simulink model "Aufgabe10_Teilsysteme"  (R2022a)
settings: Solver=ode3  StartTime=0.0  StopTime=80  FixedStep=0.01  RelTol=1e-3
undefined symbols (not defined in the file): A, I, igetr, K, MRK, PHI, Ra, sigbuilder_block, U
libraries: simulink x25
settings Model: Creator=60251  LastModifiedBy=60251

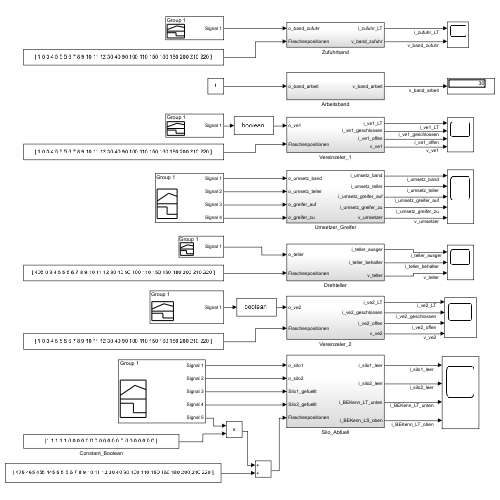
[thumbnail: Simulink's stored preview of the top-level diagram]
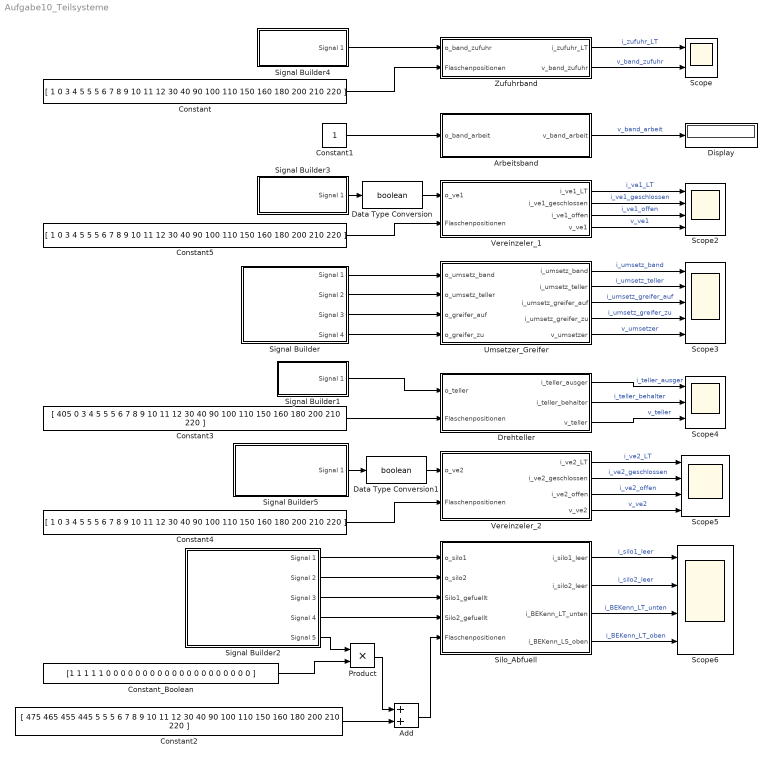
== system Aufgabe10_Teilsysteme ==
  Add : Sum
  Arbeitsband : Subsystem
  Constant : Constant  Value=[ 1 0 3 4 5 5 5 6 7 8 9 10 11 12 30 40 90 100 110 150 160 180 200 210 220 ]
  Constant1 : Constant
  Constant2 : Constant  Value=[ 475 465 455 445 5 5 5 6 7 8 9 10 11 12 30 40 90 100 110 150 160 180 200 210 220 ]
  Constant3 : Constant  Value=[ 405 0 3 4 5 5 5 6 7 8 9 10 11 12 30 40 90 100 110 150 160 180 200 210 220 ]
  Constant4 : Constant  Value=[ 1 0 3 4 5 5 5 6 7 8 9 10 11 12 30 40 90 100 110 150 160 180 200 210 220 ]
  Constant5 : Constant  Value=[ 1 0 3 4 5 5 5 6 7 8 9 10 11 12 30 40 90 100 110 150 160 180 200 210 220 ]
  Constant_Boolean : Constant  Value=[1 1 1 1 1 0 0 0 0 0 0 0 0 0 0 0 0 0 0 0 0 0 0 0 0 ]
  Data Type Conversion : DataTypeConversion  OutDataTypeStr=boolean  SaturateOnIntegerOverflow=off  RndMeth=Floor
  Data Type Conversion1 : DataTypeConversion  OutDataTypeStr=boolean  SaturateOnIntegerOverflow=off  RndMeth=Floor
  Display : Display
  Drehteller : Subsystem
  Product : Product
  Scope : Scope  NumInputPorts=2
  Scope2 : Scope  NumInputPorts=4
  Scope3 : Scope  NumInputPorts=5
  Scope4 : Scope  NumInputPorts=3
  Scope5 : Scope  NumInputPorts=4
  Scope6 : Scope  NumInputPorts=4
  Signal Builder : Subsystem  Tag=STV Subsys  LoadFcn=sigbuilder_block('load');  StartFcn=sigbuilder_block('start');  StopFcn=sigbuilder_block('stop');  ClipboardFcn=sigbuilder_block('clipboard');  mask(Sigbuilder block){tuvar=[0:10]}
      mask help: Simulink:masks:SigbuilderBlock_MD
      mask init:
      | if ~strcmp(get_param(bdroot(gcbh),'SimulationStatus'),'stopped') tuvar = sigbuilder_block('maskInit'); end
      settings: CopyFcn=sigbuilder_block('copy');  DeleteFcn=sigbuilder_block('delete');  ModelCloseFcn=sigbuilder_block('modelClose');  PreSaveFcn=sigbuilder_block('preSave');  PauseFcn=sigbuilder_block('pause');  ContinueFcn=sigbuilder_block('continue');  NameChangeFcn=sigbuilder_block('namechange');  OpenFcn=sigbuilder_block('open',[217.2 175.2 488.4 312 ]);  CloseFcn=sigbuilder_block('close');
      mask Display: plot(0, 0, 100, 100,[2, 2, 32, 32, 2], [68, 8, 8, 68, 68],[32, 2], [38, 38], [32, 19, 2],[53, 60, 44], [32, 17, 17, 2],[16, 16, 31, 31]);txt = getActiveGroup(gcbh);text(2, 100, txt,'verticalAlignment', 'top');
  Signal Builder1 : Subsystem  Tag=STV Subsys  LoadFcn=sigbuilder_block('load');  StartFcn=sigbuilder_block('start');  StopFcn=sigbuilder_block('stop');  ClipboardFcn=sigbuilder_block('clipboard');  mask(Sigbuilder block){tuvar=[0:10]}
      mask help: Simulink:masks:SigbuilderBlock_MD
      mask init:
      | if ~strcmp(get_param(bdroot(gcbh),'SimulationStatus'),'stopped') tuvar = sigbuilder_block('maskInit'); end
      settings: CopyFcn=sigbuilder_block('copy');  DeleteFcn=sigbuilder_block('delete');  ModelCloseFcn=sigbuilder_block('modelClose');  PreSaveFcn=sigbuilder_block('preSave');  PauseFcn=sigbuilder_block('pause');  ContinueFcn=sigbuilder_block('continue');  NameChangeFcn=sigbuilder_block('namechange');  OpenFcn=sigbuilder_block('open',[279 117 550.8 361.8 ]);  CloseFcn=sigbuilder_block('close');
      mask Display: plot(0, 0, 100, 100,[2, 2, 32, 32, 2], [68, 8, 8, 68, 68],[32, 2], [38, 38], [32, 19, 2],[53, 60, 44], [32, 17, 17, 2],[16, 16, 31, 31]);txt = getActiveGroup(gcbh);text(2, 100, txt,'verticalAlignment', 'top');
  Signal Builder2 : Subsystem  Tag=STV Subsys  LoadFcn=sigbuilder_block('load');  StartFcn=sigbuilder_block('start');  StopFcn=sigbuilder_block('stop');  ClipboardFcn=sigbuilder_block('clipboard');  mask(Sigbuilder block){tuvar=[0:10]}
      mask help: Simulink:masks:SigbuilderBlock_MD
      mask init:
      | if ~strcmp(get_param(bdroot(gcbh),'SimulationStatus'),'stopped') tuvar = sigbuilder_block('maskInit'); end
      settings: CopyFcn=sigbuilder_block('copy');  DeleteFcn=sigbuilder_block('delete');  ModelCloseFcn=sigbuilder_block('modelClose');  PreSaveFcn=sigbuilder_block('preSave');  PauseFcn=sigbuilder_block('pause');  ContinueFcn=sigbuilder_block('continue');  NameChangeFcn=sigbuilder_block('namechange');  OpenFcn=sigbuilder_block('open',[61.5 156.75 659.25 447 ]);  CloseFcn=sigbuilder_block('close');
      mask Display: plot(0, 0, 100, 100,[2, 2, 32, 32, 2], [68, 8, 8, 68, 68],[32, 2], [38, 38], [32, 19, 2],[53, 60, 44], [32, 17, 17, 2],[16, 16, 31, 31]);txt = getActiveGroup(gcbh);text(2, 100, txt,'verticalAlignment', 'top');
  Signal Builder3 : Subsystem  Tag=STV Subsys  LoadFcn=sigbuilder_block('load');  StartFcn=sigbuilder_block('start');  StopFcn=sigbuilder_block('stop');  ClipboardFcn=sigbuilder_block('clipboard');  mask(Sigbuilder block){tuvar=[0:10]}
      mask help: Simulink:masks:SigbuilderBlock_MD
      mask init:
      | if ~strcmp(get_param(bdroot(gcbh),'SimulationStatus'),'stopped') tuvar = sigbuilder_block('maskInit'); end
      settings: CopyFcn=sigbuilder_block('copy');  DeleteFcn=sigbuilder_block('delete');  ModelCloseFcn=sigbuilder_block('modelClose');  PreSaveFcn=sigbuilder_block('preSave');  PauseFcn=sigbuilder_block('pause');  ContinueFcn=sigbuilder_block('continue');  NameChangeFcn=sigbuilder_block('namechange');  OpenFcn=sigbuilder_block('open',[30.75 168 550.5 396 ]);  CloseFcn=sigbuilder_block('close');
      mask Display: plot(0, 0, 100, 100,[2, 2, 32, 32, 2], [68, 8, 8, 68, 68],[32, 2], [38, 38], [32, 19, 2],[53, 60, 44], [32, 17, 17, 2],[16, 16, 31, 31]);txt = getActiveGroup(gcbh);text(2, 100, txt,'verticalAlignment', 'top');
  Signal Builder4 : Subsystem  Tag=STV Subsys  LoadFcn=sigbuilder_block('load');  StartFcn=sigbuilder_block('start');  StopFcn=sigbuilder_block('stop');  ClipboardFcn=sigbuilder_block('clipboard');  mask(Sigbuilder block){tuvar=[0:10]}
      mask help: Simulink:masks:SigbuilderBlock_MD
      mask init:
      | if ~strcmp(get_param(bdroot(gcbh),'SimulationStatus'),'stopped') tuvar = sigbuilder_block('maskInit'); end
      settings: CopyFcn=sigbuilder_block('copy');  DeleteFcn=sigbuilder_block('delete');  ModelCloseFcn=sigbuilder_block('modelClose');  PreSaveFcn=sigbuilder_block('preSave');  PauseFcn=sigbuilder_block('pause');  ContinueFcn=sigbuilder_block('continue');  NameChangeFcn=sigbuilder_block('namechange');  OpenFcn=sigbuilder_block('open',[225.6 94.2 550.8 321 ]);  CloseFcn=sigbuilder_block('close');
      mask Display: plot(0, 0, 100, 100,[2, 2, 32, 32, 2], [68, 8, 8, 68, 68],[32, 2], [38, 38], [32, 19, 2],[53, 60, 44], [32, 17, 17, 2],[16, 16, 31, 31]);txt = getActiveGroup(gcbh);text(2, 100, txt,'verticalAlignment', 'top');
  Signal Builder5 : Subsystem  Tag=STV Subsys  LoadFcn=sigbuilder_block('load');  StartFcn=sigbuilder_block('start');  StopFcn=sigbuilder_block('stop');  ClipboardFcn=sigbuilder_block('clipboard');  mask(Sigbuilder block){tuvar=[0:10]}
      mask help: Simulink:masks:SigbuilderBlock_MD
      mask init:
      | if ~strcmp(get_param(bdroot(gcbh),'SimulationStatus'),'stopped') tuvar = sigbuilder_block('maskInit'); end
      settings: CopyFcn=sigbuilder_block('copy');  DeleteFcn=sigbuilder_block('delete');  ModelCloseFcn=sigbuilder_block('modelClose');  PreSaveFcn=sigbuilder_block('preSave');  PauseFcn=sigbuilder_block('pause');  ContinueFcn=sigbuilder_block('continue');  NameChangeFcn=sigbuilder_block('namechange');  OpenFcn=sigbuilder_block('open',[46.5 97.5 550.5 399.75 ]);  CloseFcn=sigbuilder_block('close');
      mask Display: plot(0, 0, 100, 100,[2, 2, 32, 32, 2], [68, 8, 8, 68, 68],[32, 2], [38, 38], [32, 19, 2],[53, 60, 44], [32, 17, 17, 2],[16, 16, 31, 31]);txt = getActiveGroup(gcbh);text(2, 100, txt,'verticalAlignment', 'top');
  Silo_Abfuell : Subsystem
  Umsetzer_Greifer : Subsystem
  Vereinzeler_1 : Subsystem
  Vereinzeler_2 : Subsystem
  Zufuhrband : Subsystem
  wires:
  Signal Builder4/1(Signal 1) -> Zufuhrband/1(o_band_zufuhr)
  Constant/1 -> Zufuhrband/2(Flaschenpositionen)
  Zufuhrband/1(i_zufuhr_LT) -> Scope/1  "i_zufuhr_LT"
  Zufuhrband/2(v_band_zufuhr) -> Scope/2  "v_band_zufuhr"
  Constant1/1 -> Arbeitsband/1(o_band_arbeit)
  Arbeitsband/1(v_band_arbeit) -> Display/1  "v_band_arbeit"
  Signal Builder3/1(Signal 1) -> Data Type Conversion/1
  Data Type Conversion/1 -> Vereinzeler_1/1(o_ve1)
  Constant5/1 -> Vereinzeler_1/2(Flaschenpositionen)
  Vereinzeler_1/1(i_ve1_LT) -> Scope2/1  "i_ve1_LT"
  Vereinzeler_1/2(i_ve1_geschlossen) -> Scope2/2  "i_ve1_geschlossen"
  Vereinzeler_1/3(i_ve1_offen) -> Scope2/3  "i_ve1_offen"
  Vereinzeler_1/4(v_ve1) -> Scope2/4  "v_ve1"
  Signal Builder/1(Signal 1) -> Umsetzer_Greifer/1(o_umsetz_band)
  Signal Builder/2(Signal 2) -> Umsetzer_Greifer/2(o_umsetz_teller)
  Signal Builder/3(Signal 3) -> Umsetzer_Greifer/3(o_greifer_auf)
  Signal Builder/4(Signal 4) -> Umsetzer_Greifer/4(o_greifer_zu)
  Umsetzer_Greifer/3(i_umsetz_greifer_auf) -> Scope3/3  "i_umsetz_greifer_auf"
  Umsetzer_Greifer/2(i_umsetz_teller) -> Scope3/2  "i_umsetz_teller"
  Umsetzer_Greifer/4(i_umsetz_greifer_zu) -> Scope3/4  "i_umsetz_greifer_zu"
  Umsetzer_Greifer/1(i_umsetz_band) -> Scope3/1  "i_umsetz_band"
  Umsetzer_Greifer/5(v_umsetzer) -> Scope3/5  "v_umsetzer"
  Drehteller/2(i_teller_behalter) -> Scope4/2  "i_teller_behalter"
  Drehteller/1(i_teller_ausger) -> Scope4/1  "i_teller_ausger"
  Drehteller/3(v_teller) -> Scope4/3  "v_teller"
  Constant3/1 -> Drehteller/2(Flaschenpositionen)
  Signal Builder1/1(Signal 1) -> Drehteller/1(o_teller)
  Vereinzeler_2/2(i_ve2_geschlossen) -> Scope5/2  "i_ve2_geschlossen"
  Vereinzeler_2/1(i_ve2_LT) -> Scope5/1  "i_ve2_LT"
  Vereinzeler_2/3(i_ve2_offen) -> Scope5/3  "i_ve2_offen"
  Vereinzeler_2/4(v_ve2) -> Scope5/4  "v_ve2"
  Signal Builder5/1(Signal 1) -> Data Type Conversion1/1
  Constant4/1 -> Vereinzeler_2/2(Flaschenpositionen)
  Data Type Conversion1/1 -> Vereinzeler_2/1(o_ve2)
  Silo_Abfuell/1(i_silo1_leer) -> Scope6/1  "i_silo1_leer"
  Silo_Abfuell/2(i_silo2_leer) -> Scope6/2  "i_silo2_leer"
  Silo_Abfuell/3(i_BEKenn_LT_unten) -> Scope6/3  "i_BEKenn_LT_unten"
  Silo_Abfuell/4(i_BEKenn_LS_oben) -> Scope6/4  "i_BEKenn_LT_oben"
  Signal Builder2/5(Signal 5) -> Product/1
  Constant_Boolean/1 -> Product/2
  Product/1 -> Add/1
  Constant2/1 -> Add/2
  Add/1 -> Silo_Abfuell/5(Flaschenpositionen)
  Signal Builder2/1(Signal 1) -> Silo_Abfuell/1(o_silo1)
  Signal Builder2/2(Signal 2) -> Silo_Abfuell/2(o_silo2)
  Signal Builder2/3(Signal 3) -> Silo_Abfuell/3(Silo1_gefuellt)
  Signal Builder2/4(Signal 4) -> Silo_Abfuell/4(Silo2_gefuellt)

== system Aufgabe10_Teilsysteme/Arbeitsband ==
  o_band_arbeit : Inport
  Gain : Gain  Gain=30
  v_band_arbeit : Outport
  wires:
  o_band_arbeit/1 -> Gain/1
  Gain/1 -> v_band_arbeit/1

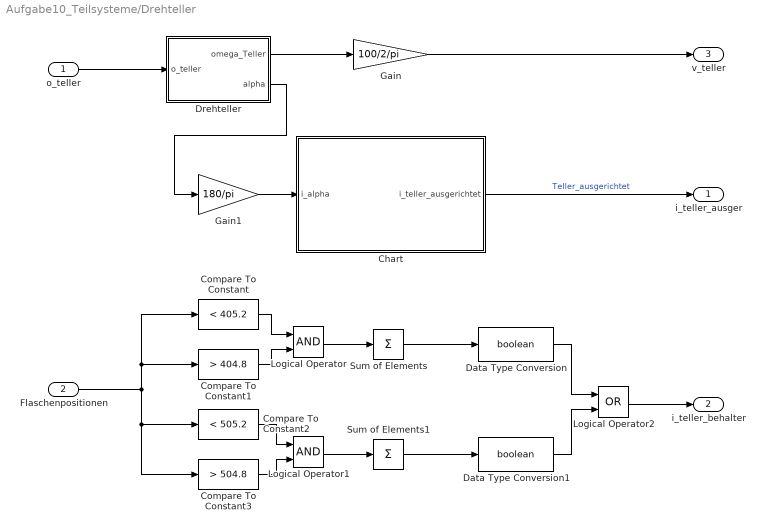
== system Aufgabe10_Teilsysteme/Drehteller ==
  o_teller : Inport
  Flaschenpositionen : Inport  Port=2
  Chart : Stateflow chart  TreatAsAtomicUnit=on
  Compare To Constant : simulink/Logic and Bit Operations/Compare To Constant  relop=<  const=405.2  OutDataTypeStr=boolean
  Compare To Constant1 : simulink/Logic and Bit Operations/Compare To Constant  relop=>  const=404.8  OutDataTypeStr=boolean
  Compare To Constant2 : simulink/Logic and Bit Operations/Compare To Constant  relop=<  const=505.2  OutDataTypeStr=boolean
  Compare To Constant3 : simulink/Logic and Bit Operations/Compare To Constant  relop=>  const=504.8  OutDataTypeStr=boolean
  Data Type Conversion : DataTypeConversion  OutDataTypeStr=boolean  SaturateOnIntegerOverflow=off  RndMeth=Floor
  Data Type Conversion1 : DataTypeConversion  OutDataTypeStr=boolean  SaturateOnIntegerOverflow=off  RndMeth=Floor
  Drehteller : Subsystem
  Gain : Gain  Gain=100/2/pi
  Gain1 : Gain  Gain=180/pi
  Logical Operator : Logic  AllPortsSameDT=off  OutDataTypeStr=boolean
  Logical Operator1 : Logic  AllPortsSameDT=off  OutDataTypeStr=boolean
  Logical Operator2 : Logic  Operator=OR  AllPortsSameDT=off  OutDataTypeStr=boolean
  Sum of Elements : Sum  Inputs=+
  Sum of Elements1 : Sum  Inputs=+
  i_teller_ausger : Outport
  i_teller_behalter : Outport  Port=2
  v_teller : Outport  Port=3
  wires:
  Compare To Constant/1 -> Logical Operator/1
  Compare To Constant1/1 -> Logical Operator/2
  Compare To Constant2/1 -> Logical Operator1/1
  Compare To Constant3/1 -> Logical Operator1/2
  Logical Operator/1 -> Sum of Elements/1
  Logical Operator1/1 -> Sum of Elements1/1
  Sum of Elements1/1 -> Data Type Conversion1/1
  Sum of Elements/1 -> Data Type Conversion/1
  Flaschenpositionen/1 -> Compare To Constant3/1, Compare To Constant2/1, Compare To Constant/1, Compare To Constant1/1
  Data Type Conversion/1 -> Logical Operator2/1
  Data Type Conversion1/1 -> Logical Operator2/2
  Logical Operator2/1 -> i_teller_behalter/1
  o_teller/1 -> Drehteller/1(o_teller)
  Drehteller/1(omega_Teller) -> Gain/1
  Gain/1 -> v_teller/1
  Chart/1(i_teller_ausgerichtet) -> i_teller_ausger/1  "Teller_ausgerichtet"
  Gain1/1 -> Chart/1(i_alpha)
  Drehteller/2(alpha) -> Gain1/1

== system Aufgabe10_Teilsysteme/Signal Builder ==
  Demux : Demux  Tag=STV Demux
      settings: DisplayOption=none
  FromWs : FromWorkspace  Tag=STV FromWs  VariableName=tuvar
      SigBuilderData=|
      | common.afterFinalStr = 'Extrapolate'
      | common.sampleTime = 0
      | dataSet.timeRange = [0 50]
      | dataSet.name = 'Group 1'
      | sbobj.Groups.Name = 'Group 1'
      | sbobj.Groups.Signals(1).Name = 'Signal 1'
      | sbobj.Groups.Signals(1).XData = [0 2 2 8 8 20.1 25 50]
      | sbobj.Groups.Signals(1).YData = [0 0 1 1 0 0 0 0]
      | sbobj.Groups.Signals(2).Name = 'Signal 2'
      | sbobj.Groups.Signals(2).XData = [0 4 5.7 5.7 7.2 7.2 20.1 20.1 25 25 50]
      | sbobj.Groups.Signals(2).YData = [0 0 0 1 1 0 0 1 1 0 0]
      | sbobj.Groups.Signals(3).Name = 'Signal 3'
      | sbobj.Groups.Signals(3).XData = [0 3 3 3.2 3.2 6 10 10 10.8 10.8 30 30 31.5 31.5 50]
      | sbobj.Groups.Signals(3).YData = [0 0 1 1 0 0 0 1 1 0 0 1 1 0 0]
      | sbobj.Groups.Signals(4).Name = 'Signal 4'
      | sbobj.Groups.Signals(4).XData = [0 4 4 5 5 6 13.7 13.7 15 15 30 30 31.5 31.5 50]
      | sbobj.Groups.Signals(4).YData = [0 0 1 1 0 0 0 1 1 0 0 1 1 0 0]
      | sbobj.Groups.TimeRange = [0 50]
  Signal 1 : Outport  Tag=STV Outport  VectorParamsAs1DForOutWhenUnconnected=off
  Signal 2 : Outport  Tag=STV Outport  Port=2  VectorParamsAs1DForOutWhenUnconnected=off
  Signal 3 : Outport  Tag=STV Outport  Port=3  VectorParamsAs1DForOutWhenUnconnected=off
  Signal 4 : Outport  Tag=STV Outport  Port=4  VectorParamsAs1DForOutWhenUnconnected=off
  wires:
  Demux/1 -> Signal 1/1
  FromWs/1 -> Demux/1
  Demux/2 -> Signal 2/1
  Demux/3 -> Signal 3/1
  Demux/4 -> Signal 4/1

== system Aufgabe10_Teilsysteme/Signal Builder1 ==
  Demux : Demux  Tag=STV Demux  Outputs=1
      settings: DisplayOption=none
  FromWs : FromWorkspace  Tag=STV FromWs  VariableName=tuvar
      SigBuilderData=|
      | common.afterFinalStr = 'Extrapolate'
      | common.sampleTime = 0
      | dataSet.timeRange = [0 50]
      | dataSet.name = 'Group 1'
      | sbobj.Groups.Name = 'Group 1'
      | sbobj.Groups.Signals.Name = 'Signal 1'
      | sbobj.Groups.Signals.XData = [0 1 1 4 6 30 30 40 40 50]
      | sbobj.Groups.Signals.YData = [0 0 1 1 1 1 0 0 1 1]
      | sbobj.Groups.TimeRange = [0 50]
  Signal 1 : Outport  Tag=STV Outport  VectorParamsAs1DForOutWhenUnconnected=off
  wires:
  Demux/1 -> Signal 1/1
  FromWs/1 -> Demux/1

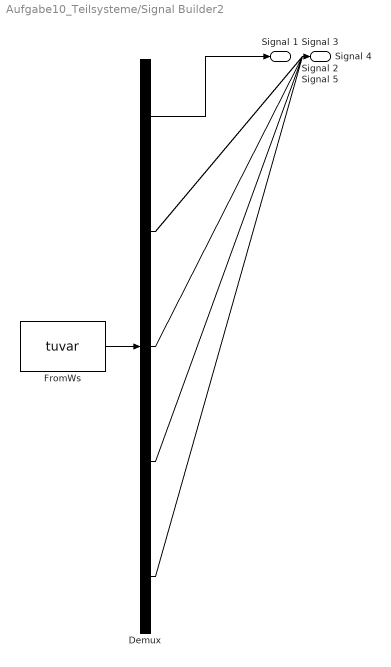
== system Aufgabe10_Teilsysteme/Signal Builder2 ==
  Demux : Demux  Tag=STV Demux  Outputs=5
      settings: DisplayOption=none
  FromWs : FromWorkspace  Tag=STV FromWs  VariableName=tuvar
      SigBuilderData=|
      | common.afterFinalStr = 'Extrapolate'
      | common.sampleTime = 0
      | dataSet.timeRange = [0 80]
      | dataSet.name = 'Group 1'
      | sbobj.Groups.Name = 'Group 1'
      | sbobj.Groups.Signals(1).Name = 'Signal 1'
      | sbobj.Groups.Signals(1).XData = [0 1 1 4 6 6 21.5 21.5 31 31 40 40 60 60 80]
      | sbobj.Groups.Signals(1).YData = [0 0 1 1 1 0 0 1 1 0 0 1 1 0 0]
      | sbobj.Groups.Signals(2).Name = 'Signal 2'
      | sbobj.Groups.Signals(2).XData = [0 1 1 6 6 40 80]
      | sbobj.Groups.Signals(2).YData = [0 0 1 1 0 0 0]
      | sbobj.Groups.Signals(3).Name = 'Signal 3'
      | sbobj.Groups.Signals(3).XData = [0 35 35 40.5 40.5 50 59.5 80]
      | sbobj.Groups.Signals(3).YData = [0 0 1 1 0 0 0 0]
      | sbobj.Groups.Signals(4).Name = 'Signal 4'
      | sbobj.Groups.Signals(4).XData = [0 50 60 80]
      | sbobj.Groups.Signals(4).YData = [0 0 0 0]
      | sbobj.Groups.Signals(5).Name = 'Signal 5'
      | sbobj.Groups.Signals(5).XData = [0 1 1 14.8 14.8 20 20 35 35 40 40 80]
      | sbobj.Groups.Signals(5).YData = [0 0 5 5 10 10 15 15 20 20 25 25]
      | sbobj.Groups.TimeRange = [0 80]
  Signal 1 : Outport  Tag=STV Outport  VectorParamsAs1DForOutWhenUnconnected=off
  Signal 2 : Outport  Tag=STV Outport  Port=2  VectorParamsAs1DForOutWhenUnconnected=off
  Signal 3 : Outport  Tag=STV Outport  Port=3  VectorParamsAs1DForOutWhenUnconnected=off
  Signal 4 : Outport  Tag=STV Outport  Port=4  VectorParamsAs1DForOutWhenUnconnected=off
  Signal 5 : Outport  Tag=STV Outport  Port=5  VectorParamsAs1DForOutWhenUnconnected=off
  wires:
  Demux/1 -> Signal 1/1
  FromWs/1 -> Demux/1
  Demux/2 -> Signal 2/1
  Demux/3 -> Signal 3/1
  Demux/4 -> Signal 4/1
  Demux/5 -> Signal 5/1

== system Aufgabe10_Teilsysteme/Signal Builder3 ==
  Demux : Demux  Tag=STV Demux  Outputs=1
      settings: DisplayOption=none
  FromWs : FromWorkspace  Tag=STV FromWs  VariableName=tuvar
      SigBuilderData=|
      | common.afterFinalStr = 'Extrapolate'
      | common.sampleTime = 0
      | dataSet.timeRange = [0 50]
      | dataSet.name = 'Group 1'
      | sbobj.Groups.Name = 'Group 1'
      | sbobj.Groups.Signals.Name = 'Signal 1'
      | sbobj.Groups.Signals.XData = [0 1 1 4 4 8.8 8.8 9 9 12.3 12.3 18.4 18.4 26.2 26.2 31.9 31.9 38.7 38.7 45 45 48.3 48.3 50]
      | sbobj.Groups.Signals.YData = [0 0 1 1 0 0 1 1 0 0 1 1 0 0 1 1 0 0 1 1 0 0 1 1]
      | sbobj.Groups.TimeRange = [0 50]
  Signal 1 : Outport  Tag=STV Outport  VectorParamsAs1DForOutWhenUnconnected=off
  wires:
  Demux/1 -> Signal 1/1
  FromWs/1 -> Demux/1

== system Aufgabe10_Teilsysteme/Signal Builder4 ==
  Demux : Demux  Tag=STV Demux  Outputs=1
      settings: DisplayOption=none
  FromWs : FromWorkspace  Tag=STV FromWs  VariableName=tuvar
      SigBuilderData=|
      | common.afterFinalStr = 'Extrapolate'
      | common.sampleTime = 0
      | dataSet.timeRange = [0 50]
      | dataSet.name = 'Group 1'
      | sbobj.Groups.Name = 'Group 1'
      | sbobj.Groups.Signals.Name = 'Signal 1'
      | sbobj.Groups.Signals.XData = [0 1 1 4 6 50]
      | sbobj.Groups.Signals.YData = [0 0 1 1 1 1]
      | sbobj.Groups.TimeRange = [0 50]
  Signal 1 : Outport  Tag=STV Outport  VectorParamsAs1DForOutWhenUnconnected=off
  wires:
  Demux/1 -> Signal 1/1
  FromWs/1 -> Demux/1

== system Aufgabe10_Teilsysteme/Signal Builder5 ==
  Demux : Demux  Tag=STV Demux  Outputs=1
      settings: DisplayOption=none
  FromWs : FromWorkspace  Tag=STV FromWs  VariableName=tuvar
      SigBuilderData=|
      | common.afterFinalStr = 'Extrapolate'
      | common.sampleTime = 0
      | dataSet.timeRange = [0 50]
      | dataSet.name = 'Group 1'
      | sbobj.Groups.Name = 'Group 1'
      | sbobj.Groups.Signals.Name = 'Signal 1'
      | sbobj.Groups.Signals.XData = [0 1 1 4 4 8.8 8.8 9 9 12.3 12.3 18.4 18.4 26.2 26.2 31.9 31.9 38.7 38.7 45 45 48.3 48.3 50]
      | sbobj.Groups.Signals.YData = [0 0 1 1 0 0 1 1 0 0 1 1 0 0 1 1 0 0 1 1 0 0 1 1]
      | sbobj.Groups.TimeRange = [0 50]
  Signal 1 : Outport  Tag=STV Outport  VectorParamsAs1DForOutWhenUnconnected=off
  wires:
  Demux/1 -> Signal 1/1
  FromWs/1 -> Demux/1

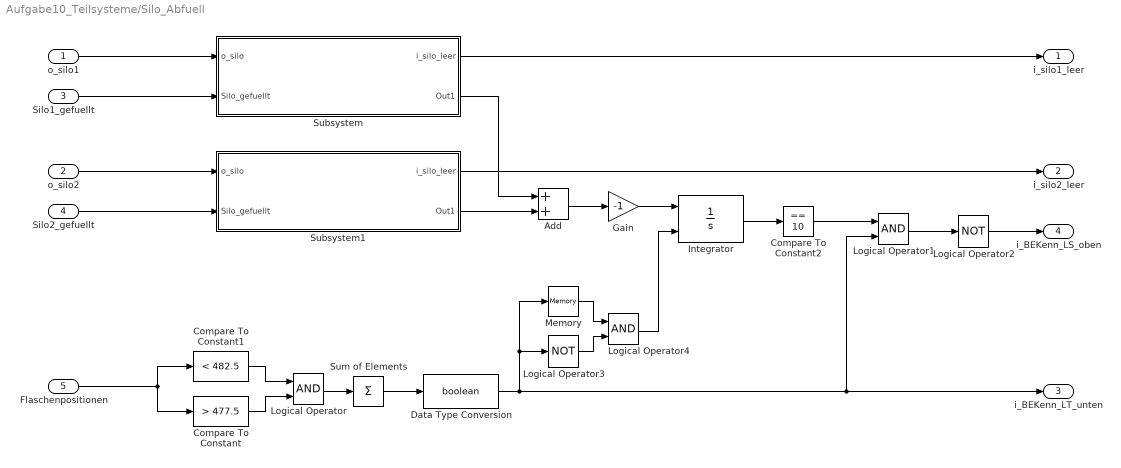
== system Aufgabe10_Teilsysteme/Silo_Abfuell ==
  o_silo1 : Inport
  o_silo2 : Inport  Port=2
  Silo1_gefuellt : Inport  Port=3
  Silo2_gefuellt : Inport  Port=4
  Flaschenpositionen : Inport  Port=5
  Add : Sum
  Compare To Constant : simulink/Logic and Bit Operations/Compare To Constant  relop=>  const=477.5  OutDataTypeStr=boolean
  Compare To Constant1 : simulink/Logic and Bit Operations/Compare To Constant  relop=<  const=482.5  OutDataTypeStr=boolean
  Compare To Constant2 : simulink/Logic and Bit Operations/Compare To Constant  relop===  const=10  OutDataTypeStr=boolean
  Data Type Conversion : DataTypeConversion  OutDataTypeStr=boolean  SaturateOnIntegerOverflow=off  RndMeth=Floor
  Gain : Gain  Gain=-1
  Integrator : Integrator  ExternalReset=rising  LimitOutput=on  UpperSaturationLimit=10  LowerSaturationLimit=0
  Logical Operator : Logic  AllPortsSameDT=off  OutDataTypeStr=boolean
  Logical Operator1 : Logic  AllPortsSameDT=off  OutDataTypeStr=boolean
  Logical Operator2 : Logic  Operator=NOT  AllPortsSameDT=off  OutDataTypeStr=boolean
  Logical Operator3 : Logic  Operator=NOT  AllPortsSameDT=off  OutDataTypeStr=boolean
  Logical Operator4 : Logic  AllPortsSameDT=off  OutDataTypeStr=boolean
  Memory : Memory
  Subsystem : Subsystem
  Subsystem1 : Subsystem
  Sum of Elements : Sum  Inputs=+
  i_silo1_leer : Outport
  i_silo2_leer : Outport  Port=2
  i_BEKenn_LT_unten : Outport  Port=3
  i_BEKenn_LS_oben : Outport  Port=4
  wires:
  o_silo1/1 -> Subsystem/1(o_silo)
  Silo1_gefuellt/1 -> Subsystem/2(Silo_gefuellt)
  Subsystem/1(i_silo_leer) -> i_silo1_leer/1
  o_silo2/1 -> Subsystem1/1(o_silo)
  Silo2_gefuellt/1 -> Subsystem1/2(Silo_gefuellt)
  Subsystem1/1(i_silo_leer) -> i_silo2_leer/1
  Compare To Constant/1 -> Logical Operator/2
  Compare To Constant1/1 -> Logical Operator/1
  Logical Operator/1 -> Sum of Elements/1
  Sum of Elements/1 -> Data Type Conversion/1
  Subsystem/2(Out1) -> Add/1
  Subsystem1/2(Out1) -> Add/2
  Add/1 -> Gain/1
  Gain/1 -> Integrator/1
  Integrator/1 -> Compare To Constant2/1
  Compare To Constant2/1 -> Logical Operator1/1
  Flaschenpositionen/1 -> Compare To Constant/1, Compare To Constant1/1
  Data Type Conversion/1 -> Logical Operator1/2, i_BEKenn_LT_unten/1, Memory/1, Logical Operator3/1
  Logical Operator1/1 -> Logical Operator2/1
  Logical Operator2/1 -> i_BEKenn_LS_oben/1
  Memory/1 -> Logical Operator4/1
  Logical Operator3/1 -> Logical Operator4/2
  Logical Operator4/1 -> Integrator/2

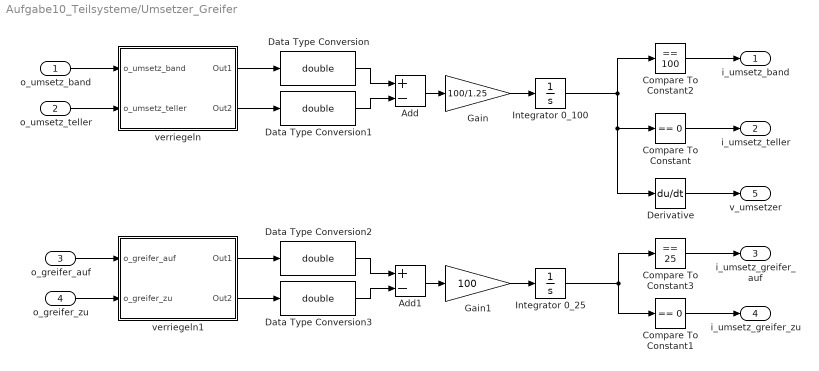
== system Aufgabe10_Teilsysteme/Umsetzer_Greifer ==
  o_umsetz_band : Inport
  o_umsetz_teller : Inport  Port=2
  o_greifer_auf : Inport  Port=3
  o_greifer_zu : Inport  Port=4
  Add : Sum  Inputs=+-
  Add1 : Sum  Inputs=+-
  Compare To Constant : simulink/Logic and Bit Operations/Compare To Constant  relop===  const=0  OutDataTypeStr=boolean
  Compare To Constant1 : simulink/Logic and Bit Operations/Compare To Constant  relop===  const=0  OutDataTypeStr=boolean
  Compare To Constant2 : simulink/Logic and Bit Operations/Compare To Constant  relop===  const=100  OutDataTypeStr=boolean
  Compare To Constant3 : simulink/Logic and Bit Operations/Compare To Constant  relop===  const=25  OutDataTypeStr=boolean
  Data Type Conversion{,1..3} (4 alike) : DataTypeConversion  OutDataTypeStr=double  SaturateOnIntegerOverflow=off  RndMeth=Floor
  Derivative : Derivative
  Gain : Gain  Gain=100/1.25
  Gain1 : Gain  Gain=100
  Integrator 0_100 : Integrator  LimitOutput=on  UpperSaturationLimit=100  LowerSaturationLimit=0
  Integrator 0_25 : Integrator  LimitOutput=on  UpperSaturationLimit=25  LowerSaturationLimit=0
  verriegeln : Subsystem
  verriegeln1 : Subsystem
  i_umsetz_band : Outport
  i_umsetz_teller : Outport  Port=2
  i_umsetz_greifer_auf : Outport  Port=3
  i_umsetz_greifer_zu : Outport  Port=4
  v_umsetzer : Outport  Port=5
  wires:
  verriegeln/2(Out2) -> Data Type Conversion1/1
  verriegeln/1(Out1) -> Data Type Conversion/1
  Data Type Conversion/1 -> Add/1
  Data Type Conversion1/1 -> Add/2
  Add/1 -> Gain/1
  Gain/1 -> Integrator 0_100/1
  Gain1/1 -> Integrator 0_25/1
  Add1/1 -> Gain1/1
  Data Type Conversion3/1 -> Add1/2
  Data Type Conversion2/1 -> Add1/1
  verriegeln1/1(Out1) -> Data Type Conversion2/1
  verriegeln1/2(Out2) -> Data Type Conversion3/1
  o_umsetz_teller/1 -> verriegeln/2(o_umsetz_teller)
  o_umsetz_band/1 -> verriegeln/1(o_umsetz_band)
  o_greifer_auf/1 -> verriegeln1/1(o_greifer_auf)
  o_greifer_zu/1 -> verriegeln1/2(o_greifer_zu)
  Integrator 0_25/1 -> Compare To Constant1/1, Compare To Constant3/1
  Compare To Constant3/1 -> i_umsetz_greifer_auf/1
  Compare To Constant1/1 -> i_umsetz_greifer_zu/1
  Integrator 0_100/1 -> Derivative/1, Compare To Constant/1, Compare To Constant2/1
  Compare To Constant/1 -> i_umsetz_teller/1
  Compare To Constant2/1 -> i_umsetz_band/1
  Derivative/1 -> v_umsetzer/1

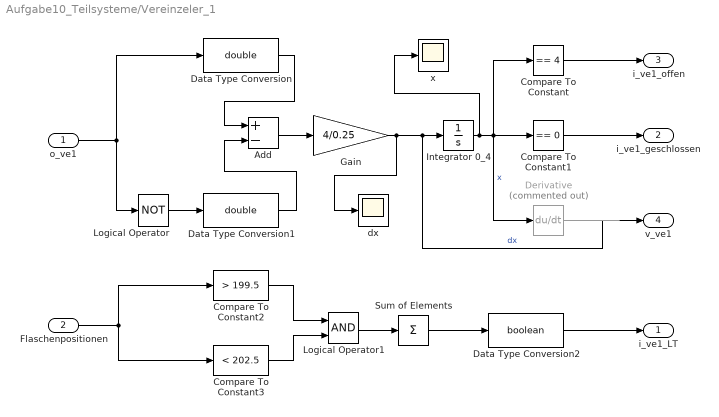
== system Aufgabe10_Teilsysteme/Vereinzeler_1 ==
  o_ve1 : Inport
  Flaschenpositionen : Inport  Port=2
  Add : Sum  Inputs=+-
  Compare To Constant : simulink/Logic and Bit Operations/Compare To Constant  relop===  const=4  OutDataTypeStr=boolean
  Compare To Constant1 : simulink/Logic and Bit Operations/Compare To Constant  relop===  const=0  OutDataTypeStr=boolean
  Compare To Constant2 : simulink/Logic and Bit Operations/Compare To Constant  relop=>  const=199.5  OutDataTypeStr=boolean
  Compare To Constant3 : simulink/Logic and Bit Operations/Compare To Constant  relop=<  const=202.5  OutDataTypeStr=boolean
  Data Type Conversion : DataTypeConversion  OutDataTypeStr=double  SaturateOnIntegerOverflow=off  RndMeth=Floor
  Data Type Conversion1 : DataTypeConversion  OutDataTypeStr=double  SaturateOnIntegerOverflow=off  RndMeth=Floor
  Data Type Conversion2 : DataTypeConversion  OutDataTypeStr=boolean  SaturateOnIntegerOverflow=off  RndMeth=Floor
  Derivative : Derivative  Commented=on
  Gain : Gain  Gain=4/0.25
  Integrator 0_4 : Integrator  LimitOutput=on  UpperSaturationLimit=4  LowerSaturationLimit=0
  Logical Operator : Logic  Operator=NOT  AllPortsSameDT=off  OutDataTypeStr=boolean
  Logical Operator1 : Logic  AllPortsSameDT=off  OutDataTypeStr=boolean
  Sum of Elements : Sum  Inputs=+
  dx : Scope
  x : Scope
  i_ve1_LT : Outport
  i_ve1_geschlossen : Outport  Port=2
  i_ve1_offen : Outport  Port=3
  v_ve1 : Outport  Port=4
  wires:
  Add/1 -> Gain/1
  Data Type Conversion/1 -> Add/1
  Data Type Conversion1/1 -> Add/2
  Logical Operator/1 -> Data Type Conversion1/1
  o_ve1/1 -> Data Type Conversion/1, Logical Operator/1
  Integrator 0_4/1 -> x/1, Derivative/1, Compare To Constant/1, Compare To Constant1/1  "x"
  Compare To Constant/1 -> i_ve1_offen/1
  Compare To Constant1/1 -> i_ve1_geschlossen/1
  Gain/1 -> dx/1, v_ve1/1, Integrator 0_4/1  "dx"
  Compare To Constant2/1 -> Logical Operator1/1
  Compare To Constant3/1 -> Logical Operator1/2
  Logical Operator1/1 -> Sum of Elements/1
  Flaschenpositionen/1 -> Compare To Constant3/1, Compare To Constant2/1
  Sum of Elements/1 -> Data Type Conversion2/1
  Data Type Conversion2/1 -> i_ve1_LT/1
  Derivative/1 -> ?

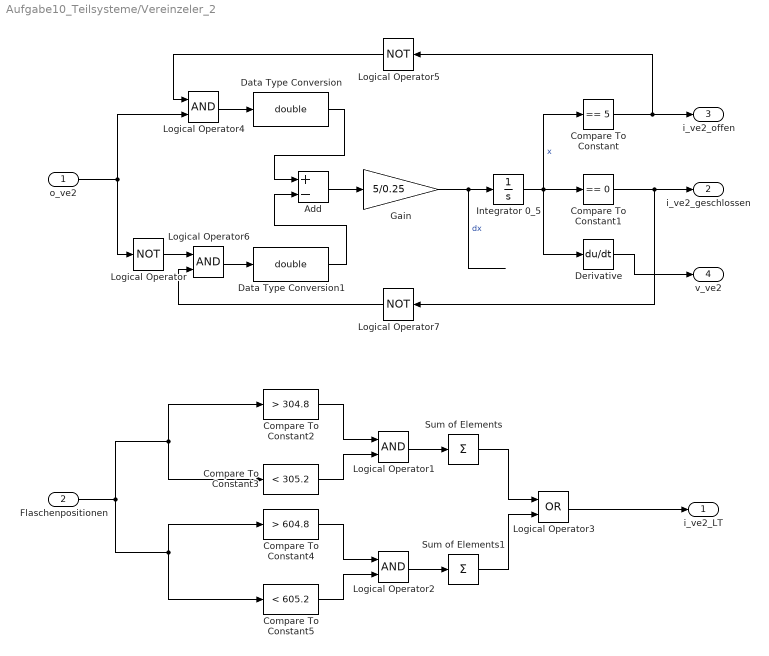
== system Aufgabe10_Teilsysteme/Vereinzeler_2 ==
  o_ve2 : Inport
  Flaschenpositionen : Inport  Port=2
  Add : Sum  Inputs=+-
  Compare To Constant : simulink/Logic and Bit Operations/Compare To Constant  relop===  const=5  OutDataTypeStr=boolean
  Compare To Constant1 : simulink/Logic and Bit Operations/Compare To Constant  relop===  const=0  OutDataTypeStr=boolean
  Compare To Constant2 : simulink/Logic and Bit Operations/Compare To Constant  relop=>  const=304.8  OutDataTypeStr=boolean
  Compare To Constant3 : simulink/Logic and Bit Operations/Compare To Constant  relop=<  const=305.2  OutDataTypeStr=boolean
  Compare To Constant4 : simulink/Logic and Bit Operations/Compare To Constant  relop=>  const=604.8  OutDataTypeStr=boolean
  Compare To Constant5 : simulink/Logic and Bit Operations/Compare To Constant  relop=<  const=605.2  OutDataTypeStr=boolean
  Data Type Conversion : DataTypeConversion  OutDataTypeStr=double  SaturateOnIntegerOverflow=off  RndMeth=Floor
  Data Type Conversion1 : DataTypeConversion  OutDataTypeStr=double  SaturateOnIntegerOverflow=off  RndMeth=Floor
  Derivative : Derivative
  Gain : Gain  Gain=5/0.25
  Integrator 0_5 : Integrator  LimitOutput=on  UpperSaturationLimit=5  LowerSaturationLimit=0
  Logical Operator : Logic  Operator=NOT  AllPortsSameDT=off  OutDataTypeStr=boolean
  Logical Operator{1..2,4,6} (4 alike) : Logic  AllPortsSameDT=off  OutDataTypeStr=boolean
  Logical Operator3 : Logic  Operator=OR  AllPortsSameDT=off  OutDataTypeStr=boolean
  Logical Operator5 : Logic  Operator=NOT  AllPortsSameDT=off  OutDataTypeStr=boolean
  Logical Operator7 : Logic  Operator=NOT  AllPortsSameDT=off  OutDataTypeStr=boolean
  Sum of Elements : Sum  Inputs=+
  Sum of Elements1 : Sum  Inputs=+
  i_ve2_LT : Outport
  i_ve2_geschlossen : Outport  Port=2
  i_ve2_offen : Outport  Port=3
  v_ve2 : Outport  Port=4
  wires:
  Logical Operator3/1 -> i_ve2_LT/1
  Sum of Elements/1 -> Logical Operator3/1
  Logical Operator1/1 -> Sum of Elements/1
  Compare To Constant3/1 -> Logical Operator1/2
  Compare To Constant2/1 -> Logical Operator1/1
  Gain/1 -> Integrator 0_5/1  "dx"
  Compare To Constant1/1 -> Logical Operator7/1, i_ve2_geschlossen/1
  Compare To Constant/1 -> Logical Operator5/1, i_ve2_offen/1
  Integrator 0_5/1 -> Derivative/1, Compare To Constant1/1, Compare To Constant/1  "x"
  o_ve2/1 -> Logical Operator4/2, Logical Operator/1
  Logical Operator/1 -> Logical Operator6/1
  Data Type Conversion1/1 -> Add/2
  Data Type Conversion/1 -> Add/1
  Add/1 -> Gain/1
  Compare To Constant4/1 -> Logical Operator2/1
  Compare To Constant5/1 -> Logical Operator2/2
  Logical Operator2/1 -> Sum of Elements1/1
  Flaschenpositionen/1 -> Compare To Constant3/1, Compare To Constant2/1, Compare To Constant5/1, Compare To Constant4/1
  Sum of Elements1/1 -> Logical Operator3/2
  Logical Operator4/1 -> Data Type Conversion/1
  Logical Operator6/1 -> Data Type Conversion1/1
  Logical Operator7/1 -> Logical Operator6/2
  Logical Operator5/1 -> Logical Operator4/1
  Derivative/1 -> v_ve2/1

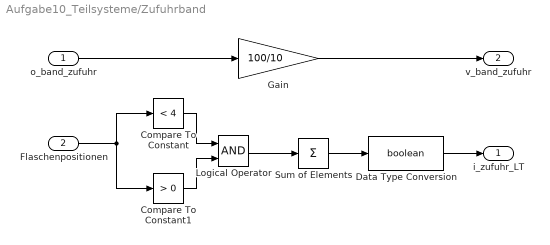
== system Aufgabe10_Teilsysteme/Zufuhrband ==
  o_band_zufuhr : Inport
  Flaschenpositionen : Inport  Port=2
  Compare To Constant : simulink/Logic and Bit Operations/Compare To Constant  relop=<  const=4  OutDataTypeStr=boolean
  Compare To Constant1 : simulink/Logic and Bit Operations/Compare To Constant  relop=>  const=0  OutDataTypeStr=boolean
  Data Type Conversion : DataTypeConversion  OutDataTypeStr=boolean  SaturateOnIntegerOverflow=off  RndMeth=Floor
  Gain : Gain  Gain=100/10
  Logical Operator : Logic  AllPortsSameDT=off  OutDataTypeStr=boolean
  Sum of Elements : Sum  Inputs=+
  i_zufuhr_LT : Outport
  v_band_zufuhr : Outport  Port=2
  wires:
  Flaschenpositionen/1 -> Compare To Constant1/1, Compare To Constant/1
  Compare To Constant/1 -> Logical Operator/1
  Compare To Constant1/1 -> Logical Operator/2
  Logical Operator/1 -> Sum of Elements/1
  Sum of Elements/1 -> Data Type Conversion/1
  Data Type Conversion/1 -> i_zufuhr_LT/1
  o_band_zufuhr/1 -> Gain/1
  Gain/1 -> v_band_zufuhr/1

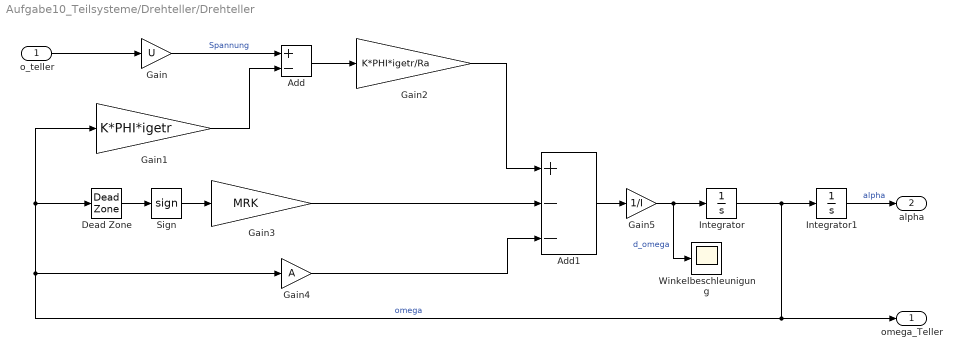
== system Aufgabe10_Teilsysteme/Drehteller/Drehteller ==
  o_teller : Inport
  Add : Sum  Inputs=+-
  Add1 : Sum  Inputs=+--
  Dead Zone : DeadZone
  Gain : Gain  Gain=U
  Gain1 : Gain  Gain=K*PHI*igetr
  Gain2 : Gain  Gain=K*PHI*igetr/Ra
  Gain3 : Gain  Gain=MRK
  Gain4 : Gain  Gain=A
  Gain5 : Gain  Gain=1/I
  Integrator : Integrator
  Integrator1 : Integrator
  Sign : Signum
  Winkelbeschleunigung : Scope
  omega_Teller : Outport
  alpha : Outport  Port=2
  wires:
  Add1/1 -> Gain5/1
  Sign/1 -> Gain3/1
  Add/1 -> Gain2/1
  Dead Zone/1 -> Sign/1
  Integrator1/1 -> alpha/1  "alpha"
  Gain1/1 -> Add/2
  Gain2/1 -> Add1/1
  Gain5/1 -> Winkelbeschleunigung/1, Integrator/1  "d_omega"
  Gain3/1 -> Add1/2
  Gain4/1 -> Add1/3
  o_teller/1 -> Gain/1
  Gain/1 -> Add/1  "Spannung"
  Integrator/1 -> omega_Teller/1, Dead Zone/1, Gain1/1, Gain4/1, Integrator1/1  "omega"

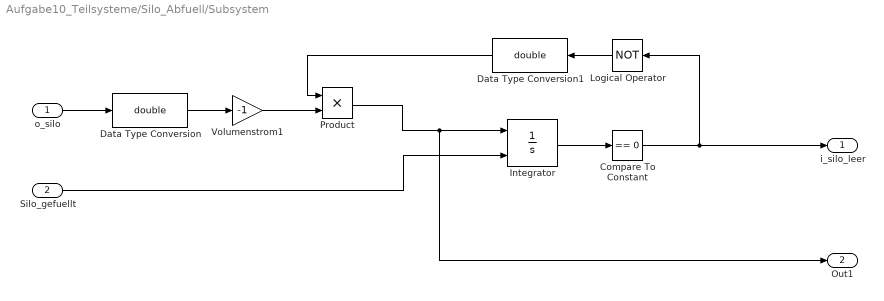
== system Aufgabe10_Teilsysteme/Silo_Abfuell/Subsystem ==
  o_silo : Inport
  Silo_gefuellt : Inport  Port=2
  Compare To Constant : simulink/Logic and Bit Operations/Compare To Constant  relop===  const=0  OutDataTypeStr=boolean
  Data Type Conversion : DataTypeConversion  OutDataTypeStr=double  SaturateOnIntegerOverflow=off  RndMeth=Floor
  Data Type Conversion1 : DataTypeConversion  OutDataTypeStr=double  SaturateOnIntegerOverflow=off  RndMeth=Floor
  Integrator : Integrator  ExternalReset=rising  InitialCondition=10  LimitOutput=on  UpperSaturationLimit=10  LowerSaturationLimit=0
  Logical Operator : Logic  Operator=NOT  AllPortsSameDT=off  OutDataTypeStr=boolean
  Product : Product
  Volumenstrom1 : Gain  Gain=-1
  i_silo_leer : Outport
  Out1 : Outport  Port=2
  wires:
  Logical Operator/1 -> Data Type Conversion1/1
  Data Type Conversion1/1 -> Product/1
  Integrator/1 -> Compare To Constant/1
  Compare To Constant/1 -> Logical Operator/1, i_silo_leer/1
  Product/1 -> Out1/1, Integrator/1
  Volumenstrom1/1 -> Product/2
  Data Type Conversion/1 -> Volumenstrom1/1
  Silo_gefuellt/1 -> Integrator/2
  o_silo/1 -> Data Type Conversion/1

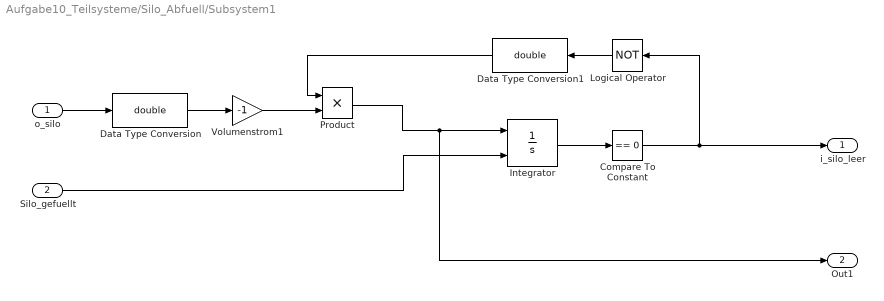
== system Aufgabe10_Teilsysteme/Silo_Abfuell/Subsystem1 ==
  o_silo : Inport
  Silo_gefuellt : Inport  Port=2
  Compare To Constant : simulink/Logic and Bit Operations/Compare To Constant  relop===  const=0  OutDataTypeStr=boolean
  Data Type Conversion : DataTypeConversion  OutDataTypeStr=double  SaturateOnIntegerOverflow=off  RndMeth=Floor
  Data Type Conversion1 : DataTypeConversion  OutDataTypeStr=double  SaturateOnIntegerOverflow=off  RndMeth=Floor
  Integrator : Integrator  ExternalReset=rising  InitialCondition=10  LimitOutput=on  UpperSaturationLimit=10  LowerSaturationLimit=0
  Logical Operator : Logic  Operator=NOT  AllPortsSameDT=off  OutDataTypeStr=boolean
  Product : Product
  Volumenstrom1 : Gain  Gain=-1
  i_silo_leer : Outport
  Out1 : Outport  Port=2
  wires:
  o_silo/1 -> Data Type Conversion/1
  Silo_gefuellt/1 -> Integrator/2
  Data Type Conversion/1 -> Volumenstrom1/1
  Volumenstrom1/1 -> Product/2
  Product/1 -> Integrator/1, Out1/1
  Compare To Constant/1 -> i_silo_leer/1, Logical Operator/1
  Integrator/1 -> Compare To Constant/1
  Data Type Conversion1/1 -> Product/1
  Logical Operator/1 -> Data Type Conversion1/1

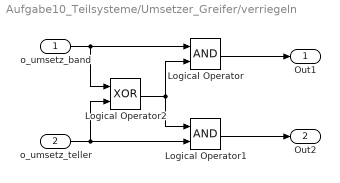
== system Aufgabe10_Teilsysteme/Umsetzer_Greifer/verriegeln ==
  o_umsetz_band : Inport
  o_umsetz_teller : Inport  Port=2
  Logical Operator : Logic  AllPortsSameDT=off  OutDataTypeStr=boolean
  Logical Operator1 : Logic  AllPortsSameDT=off  OutDataTypeStr=boolean
  Logical Operator2 : Logic  Operator=XOR  AllPortsSameDT=off  OutDataTypeStr=boolean
  Out1 : Outport
  Out2 : Outport  Port=2
  wires:
  Logical Operator1/1 -> Out2/1
  Logical Operator/1 -> Out1/1
  o_umsetz_band/1 -> Logical Operator/1, Logical Operator2/1
  o_umsetz_teller/1 -> Logical Operator2/2, Logical Operator1/2
  Logical Operator2/1 -> Logical Operator1/1, Logical Operator/2

== system Aufgabe10_Teilsysteme/Umsetzer_Greifer/verriegeln1 ==
  o_greifer_auf : Inport
  o_greifer_zu : Inport  Port=2
  Logical Operator : Logic  AllPortsSameDT=off  OutDataTypeStr=boolean
  Logical Operator1 : Logic  AllPortsSameDT=off  OutDataTypeStr=boolean
  Logical Operator2 : Logic  Operator=XOR  AllPortsSameDT=off  OutDataTypeStr=boolean
  Out1 : Outport
  Out2 : Outport  Port=2
  wires:
  Logical Operator2/1 -> Logical Operator/2, Logical Operator1/1
  o_greifer_zu/1 -> Logical Operator1/2, Logical Operator2/2
  o_greifer_auf/1 -> Logical Operator2/1, Logical Operator/1
  Logical Operator/1 -> Out1/1
  Logical Operator1/1 -> Out2/1

== stateflow chart Aufgabe10_Teilsysteme/Drehteller/Chart ==
  state ausgerichtet
    en:i_teller_ausgerichtet=1
  state eingerichtet
    en:i_teller_ausgerichtet=0
  (default) -> ausgerichtet
  eingerichtet -> ausgerichtet : [mod(i_alpha+1,90)<=2]
  ausgerichtet -> eingerichtet : [mod(i_alpha+1,90)>2]
  data: i_alpha input; i_teller_ausgerichtet output
